simulink model "AcousticNoiseCancellationDSKC6713"  (Simulink 6.5)
settings: Solver=FixedStepDiscrete  StartTime=0.0  StopTime=inf  RelTol=1e-3
PreLoadFcn:
  | load dspwlets;
PostLoadFcn:
  | c6000demoscallback
undefined symbols (not defined in the file or in its folder): bit
libraries: c6713dsklib x4, c6000tgtpreflib x1, dspsigops x1, dspadpt3 x1, dspbioslib x1
CloseFcn:
  | clear fs hid hir lod lor noisdopp ts;
settings Model: RequirementInfo=9  Creator=don  LastModifiedBy=Administrator  CovMetricSettings=d  ExtModeTrigMode=oneshot  ExtModeArmWhenConnect=off  ProdHWDeviceType=TI C6000
settings SolverCC: PositivePriorityOrder=on
settings DataIOCC: LimitDataPoints=off  SaveOutput=off  SaveTime=off  SignalLoggingName=sigsOut
settings OptimizationCC: BlockReduction=off  BooleanDataType=off  InlineParams=on  InlineInvariantSignals=on  RollThreshold=2  OptimizeModelRefInitCode=on  LifeSpan=1  BufferReusableBoundary=off
settings DebuggingCC: CheckExecutionContextPreStartOutputMsg=on  CheckExecutionContextRuntimeOutputMsg=on  SolverPrmCheckMsg=none  InheritedTsInSrcMsg=none  MultiTaskDSMMsg=warning  MultiTaskCondExecSysMsg=none  IntegerOverflowMsg=none  StrictBusMsg=None
settings HardwareCC: ProdBitPerLong=40  ProdIntDivRoundTo=Zero  ProdEndianess=LittleEndian  ProdHWDeviceType=TI C6000  TargetHWDeviceType=32-bit Generic
settings ModelReferenceCC: UpdateModelReferenceTargets=IfOutOfDate
settings RTWCC: SystemTargetFile=ti_c6000_ert.tlc  GenCodeOnly=on  TemplateMakefile=ti_c6000_ert.tmf  ProcessScript=ti_c6000_ert_make_rtw_hook  IncludeERTFirstTime=on
settings CodeAppCC: IgnoreCustomStorageClasses=off  PrefixModelToSubsysFcnNames=off  CustomSymbolStrFcn=$F$N$M
settings C6000ERTTargetCC: TargetFcnLib=ansi_tfl_tmw.mat  GenFloatMathFcnCalls=ANSI_C  UtilityFuncGeneration=Auto  GenerateFullHeader=on  GenerateSampleERTMain=on  GenerateTestInterfaces=off  IsPILTarget=off  ModelReferenceCompliant=off  IncludeMdlTerminateFcn=on  CombineOutputUpdateFcns=on  SuppressErrorStatus=off  IncludeFileDelimiter=Auto  ERTCustomFileBanners=on  SupportAbsoluteTime=on  LogVarNameModifier=rt_  MatFileLogging=off  MultiInstanceERTCode=off  SupportNonFinite=on  SupportComplex=on  PurelyIntegerCode=off  SupportContinuousTime=on  SupportNonInlinedSFcns=on  EnableShiftOperators=on  ParenthesesLevel=Nominal  GenerateErtSFunction=off  GenerateASAP2=off  ExtMode=off  ExtModeTransport=0  ExtModeStaticAlloc=off  ExtModeStaticAllocSize=1000000  ExtModeTesting=off  ExtModeMexFile=ext_comm  InlinedParameterPlacement=NonHierarchical  TargetOS=BareBoardExample  MultiInstanceErrorCode=Error  RateGroupingCode=on  RootIOFormat=Individual arguments  RTWCAPISignals=off  RTWCAPIParams=off  RTWCAPIStates=off  ERTSrcFileBannerTemplate=ert_code_template.cgt  ERTHdrFileBannerTemplate=ert_code_template.cgt  ERTDataSrcFileTemplate=ert_code_template.cgt  ERTDataHdrFileTemplate=ert_code_template.cgt  ERTCustomFileTemplate=example_file_process.tlc  ModuleNamingRule=Unspecified  SignalDisplayLevel=10  ParamTuneLevel=10  GlobalDataDefinition=Auto  DataDefinitionFile=global.c  GlobalDataReference=Auto  DataReferenceFile=global.h  GRTInterface=off  EnableUserReplacementTypes=off  MemSecPackage=--- None ---  MemSecDataConstants=Default  MemSecDataIO=Default  MemSecDataInternal=Default  MemSecDataParameters=Default  MemSecFuncInitTerm=Default  MemSecFuncExecute=Default  exportCCSObj=on  ccsObjName=CCS_Obj  useDSPBIOS=on  ProfileGenCode=off  InlineDSPBlks=on  FPopt=off  memModel=Far_Aggregate  optLevel=Function(-o2)  CompilerVerbosity=Quiet  InterruptThreshOnC6x=off  SymbolicDebugOnC6x=off  RetainAsmFiles=off  RetainObjFiles=on  CreateMapFile=on  UserStackSize=8192  c6000BuildAction=Build_and_execute  OverrunAction=Notify_and_continue  OverrunNotificationMethod=Turn_on_LEDs

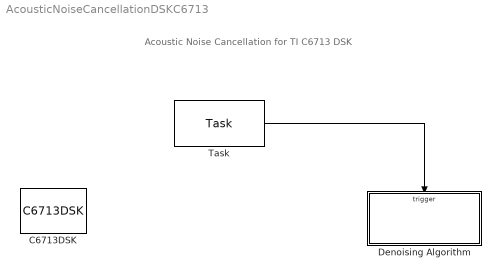
== system AcousticNoiseCancellationDSKC6713 ==
  note: Acoustic Noise Cancellation for TI C6713 DSK
  C6713DSK : c6000tgtpreflib/C6713DSK  Tag=C6000 TARGET PREFERENCES BLOCK  SystemSampleTime=-1
  Denoising Algorithm : Subsystem  TreatAsAtomicUnit=on
  Task : dspbioslib/Task  SystemSampleTime=-1  taskName=Task0  taskPriority=1  taskExecutionOrder=1  taskStackSize=4096  stackMemSegment=IRAM  monitorStackUse=off  taskYield=off  parentmanaget=on  tickres=1/1000  ticklen=32bits  taskTrigger=off
  wires:
  Task/1 -> Denoising Algorithm/Trigger

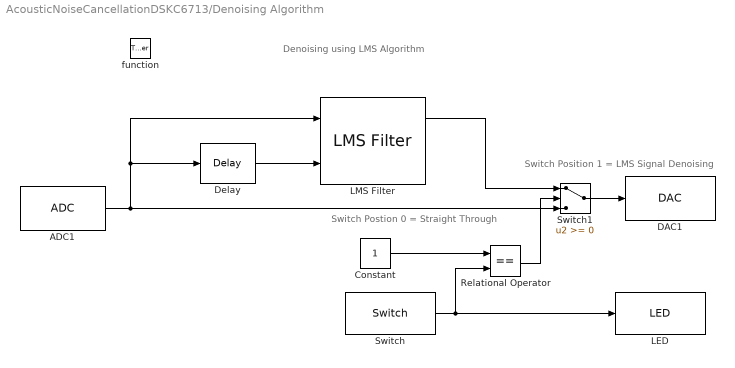
== system AcousticNoiseCancellationDSKC6713/Denoising Algorithm ==
  note: Denoising using LMS Algorithm
  note: Switch Postion 0 = Straight Through
  note: Switch Position 1 = LMS Signal Denoising
  function : TriggerPort  TriggerType=function-call
  ADC1 : c6713dsklib/ADC  ADCsource=Mic In  MicGain=on  Stereo=off  SampleRate=48 kHz  CodecDataFormat=16-bit  OutputDataType=Single  Scaling=Normalize  SourceGain=0.0  FrameSize=64  inheritSampleTime=on
  Constant : Constant  Value=1  OutDataTypeMode=int16  OutDataType=sfix(16)  ConRadixGroup=Use specified scaling  OutScaling=2^0  SampleTime=inf  FramePeriod=inf
  DAC1 : c6713dsklib/DAC  CodecDataFormat=16-bit  SampleRate=48 kHz  Scaling=Normalize  DacAtten=0.0  OverflowMode=Wrap
  Delay : dspsigops/Delay  dly_unit=Frames  delay=1  ic_detail=off  dif_ic_for_ch=off  dif_ic_for_dly=off  ic=0  reset_popup=None
  LED : c6713dsklib/LED
  LMS Filter : dspadpt3/LMS Filter  DialogController=dspDDGCreate  DialogControllerArgs=DataTag1  Algo=LMS  L=32  stepflag=Dialog  mu=0.005  leakage=1.0  ic=0  Adapt=off  resetflag=None  weights=off  secondCoeffMode=User-defined  secondCoeffWordLength=2  secondCoeffFracLength=15  accum2Mode=User-defined  accum2FracLength=20  prodOutput2Mode=User-defined  prodOutput2FracLength=20  prodOutput3Mode=User-defined  prodOutput3FracLength=20  prodOutput4Mode=User-defined  prodOutput4FracLength=20  quotientMode=User-defined  quotientFracLength=20  roundingMode=Floor  overflowMode=off  addnparflag=off
  Relational Operator : RelationalOperator  Operator===  LogicOutDataTypeMode=Boolean
  Switch : c6713dsklib/Switch  sw0=on  sw1=on  sw2=on  sw3=on  dType=Integer  Ts=-1
  Switch1 : Switch
  wires:
  ADC1/1 -> LMS Filter/1, Delay/1, Switch1/3
  Switch1/1 -> DAC1/1
  Constant/1 -> Relational Operator/1
  Switch/1 -> Relational Operator/2, LED/1
  Relational Operator/1 -> Switch1/2
  Delay/1 -> LMS Filter/2
  LMS Filter/1 -> Switch1/1
